simulink model "Tx_Rx"  (R2020a)
settings: Solver=VariableStepAuto  StartTime=0.0  StopTime=640e-9  RelTol=1e-3
libraries: msbUtilities x102, simulink_extras x15, dspswit3 x4, dspsigops x2
(part 3 of 3)

== matlab function Tx_Rx/BER_calculator/PI&PS/Phase Interpolator/MATLAB Function ==
  data: LSB_4bit input; c0_0 output; clk_s1 input; clk_s3 input; c0_1 output; c1_0 output; c1_1 output; c2_0 output; c2_1 output; c3_0 output; c3_1 output; c4_0 output; c4_1 output; c5_0 output; c5_1 output; c6_0 output; c6_1 output; c7_0 output; c7_1 output; c8_0 output; c8_1 output; c9_0 output; c9_1 output; c10_0 output; c10_1 output; c11_0 output; c11_1 output; c12_0 output; c12_1 output; c13_0 output; c13_1 output; c14_0 output; c14_1 output; c15_0 output; c15_1 output
function [c0_0,c0_1,c1_0,c1_1,c2_0,c2_1,c3_0,c3_1,c4_0,c4_1,c5_0,c5_1,c6_0,c6_1,c7_0,c7_1,c8_0,c8_1,c9_0,c9_1,c10_0,c10_1,c11_0,c11_1,c12_0,c12_1,c13_0,c13_1,c14_0,c14_1,c15_0,c15_1] = phase_interpolator(LSB_4bit,clk_s1,clk_s3)
    switch LSB_4bit
        case 0
            c0_0 = clk_s1;
            c0_1 = clk_s3;
            c1_0 = 0;
            c1_1 = 0;
            c2_0 = 0;
            c2_1 = 0;
            c3_0 = 0;
            c3_1 = 0;
            c4_0 = 0;
            c4_1 = 0;
            c5_0 = 0;
            c5_1 = 0;
            c6_0 = 0;
            c6_1 = 0;
            c7_0 = 0;
            c7_1 = 0;
            c8_0 = 0;
            c8_1 = 0;
            c9_0 = 0;
            c9_1 = 0;
            c10_0 = 0;
            c10_1 = 0;
            c11_0 = 0;
            c11_1 = 0;
            c12_0 = 0;
            c12_1 = 0;
            c13_0 = 0;
            c13_1 = 0;
            c14_0 = 0;
            c14_1 = 0;
            c15_0 = 0;
            c15_1 = 0;
        case 1
            c0_0 = 0;
            c0_1 = 0;
            c1_0 = clk_s1;
            c1_1 = clk_s3;
            c2_0 = 0;
            c2_1 = 0;
            c3_0 = 0;
            c3_1 = 0;
            c4_0 = 0;
            c4_1 = 0;
            c5_0 = 0;
            c5_1 = 0;
            c6_0 = 0;
            c6_1 = 0;
            c7_0 = 0;
            c7_1 = 0;
            c8_0 = 0;
            c8_1 = 0;
            c9_0 = 0;
            c9_1 = 0;
            c10_0 = 0;
            c10_1 = 0;
            c11_0 = 0;
            c11_1 = 0;
            c12_0 = 0;
            c12_1 = 0;
            c13_0 = 0;
            c13_1 = 0;
            c14_0 = 0;
            c14_1 = 0;
            c15_0 = 0;
            c15_1 = 0;
        case 10
            c0_0 = 0;
            c0_1 = 0;
            c1_0 = 0;
            c1_1 = 0;
            c2_0 = clk_s1;
            c2_1 = clk_s3;
            c3_0 = 0;
            c3_1 = 0;
            c4_0 = 0;
            c4_1 = 0;
            c5_0 = 0;
            c5_1 = 0;
            c6_0 = 0;
            c6_1 = 0;
            c7_0 = 0;
            c7_1 = 0;
            c8_0 = 0;
            c8_1 = 0;
            c9_0 = 0;
            c9_1 = 0;
            c10_0 = 0;
            c10_1 = 0;
            c11_0 = 0;
            c11_1 = 0;
            c12_0 = 0;
            c12_1 = 0;
            c13_0 = 0;
            c13_1 = 0;
            c14_0 = 0;
            c14_1 = 0;
            c15_0 = 0;
            c15_1 = 0;
        case 11
            c0_0 = 0;
            c0_1 = 0;
            c1_0 = 0;
            c1_1 = 0;
            c2_0 = 0;
            c2_1 = 0;
            c3_0 = clk_s1;
            c3_1 = clk_s3;
            c4_0 = 0;
            c4_1 = 0;
            c5_0 = 0;
            c5_1 = 0;
            c6_0 = 0;
            c6_1 = 0;
            c7_0 = 0;
            c7_1 = 0;
            c8_0 = 0;
            c8_1 = 0;
            c9_0 = 0;
            c9_1 = 0;
            c10_0 = 0;
            c10_1 = 0;
            c11_0 = 0;
            c11_1 = 0;
            c12_0 = 0;
            c12_1 = 0;
            c13_0 = 0;
            c13_1 = 0;
            c14_0 = 0;
            c14_1 = 0;
            c15_0 = 0;
            c15_1 = 0;
        case 100
            c0_0 = 0;
            c0_1 = 0;
            c1_0 = 0;
            c1_1 = 0;
            c2_0 = 0;
            c2_1 = 0;
            c3_0 = 0;
            c3_1 = 0;
            c4_0 = clk_s1;
            c4_1 = clk_s3;
            c5_0 = 0;
            c5_1 = 0;
            c6_0 = 0;
            c6_1 = 0;
            c7_0 = 0;
            c7_1 = 0;
            c8_0 = 0;
            c8_1 = 0;
            c9_0 = 0;
            c9_1 = 0;
            c10_0 = 0;
            c10_1 = 0;
            c11_0 = 0;
            c11_1 = 0;
            c12_0 = 0;
            c12_1 = 0;
            c13_0 = 0;
            c13_1 = 0;
            c14_0 = 0;
            c14_1 = 0;
            c15_0 = 0;
            c15_1 = 0;
        case 101
            c0_0 = 0;
            c0_1 = 0;
            c1_0 = 0;
            c1_1 = 0;
            c2_0 = 0;
            c2_1 = 0;
            c3_0 = 0;
            c3_1 = 0;
            c4_0 = 0;
            c4_1 = 0;
            c5_0 = clk_s1;
            c5_1 = clk_s3;
            c6_0 = 0;
            c6_1 = 0;
            c7_0 = 0;
            c7_1 = 0;
            c8_0 = 0;
            c8_1 = 0;
            c9_0 = 0;
            c9_1 = 0;
            c10_0 = 0;
            c10_1 = 0;
            c11_0 = 0;
            c11_1 = 0;
            c12_0 = 0;
            c12_1 = 0;
            c13_0 = 0;
            c13_1 = 0;
            c14_0 = 0;
            c14_1 = 0;
            c15_0 = 0;
            c15_1 = 0;
        case 110
            c0_0 = 0;
            c0_1 = 0;
            c1_0 = 0;
            c1_1 = 0;
            c2_0 = 0;
            c2_1 = 0;
            c3_0 = 0;
            c3_1 = 0;
            c4_0 = 0;
            c4_1 = 0;
            c5_0 = 0;
            c5_1 = 0;
            c6_0 = clk_s1;
            c6_1 = clk_s3;
            c7_0 = 0;
            c7_1 = 0;
            c8_0 = 0;
            c8_1 = 0;
            c9_0 = 0;
            c9_1 = 0;
            c10_0 = 0;
            c10_1 = 0;
            c11_0 = 0;
            c11_1 = 0;
            c12_0 = 0;
            c12_1 = 0;
            c13_0 = 0;
            c13_1 = 0;
            c14_0 = 0;
            c14_1 = 0;
            c15_0 = 0;
            c15_1 = 0;
        case 111
            c0_0 = 0;
            c0_1 = 0;
            c1_0 = 0;
            c1_1 = 0;
            c2_0 = 0;
            c2_1 = 0;
            c3_0 = 0;
            c3_1 = 0;
            c4_0 = 0;
            c4_1 = 0;
            c5_0 = 0;
            c5_1 = 0;
            c6_0 = 0;
            c6_1 = 0;
            c7_0 = clk_s1;
            c7_1 = clk_s3;
            c8_0 = 0;
            c8_1 = 0;
            c9_0 = 0;
            c9_1 = 0;
            c10_0 = 0;
            c10_1 = 0;
            c11_0 = 0;
            c11_1 = 0;
            c12_0 = 0;
            c12_1 = 0;
            c13_0 = 0;
            c13_1 = 0;
            c14_0 = 0;
            c14_1 = 0;
            c15_0 = 0;
            c15_1 = 0;
        case 1000
            c0_0 = 0;
            c0_1 = 0;
            c1_0 = 0;
            c1_1 = 0;
            c2_0 = 0;
            c2_1 = 0;
            c3_0 = 0;
            c3_1 = 0;
            c4_0 = 0;
            c4_1 = 0;
            c5_0 = 0;
            c5_1 = 0;
            c6_0 = 0;
            c6_1 = 0;
            c7_0 = 0;
            c7_1 = 0;
            c8_0 = clk_s1;
            c8_1 = clk_s3;
            c9_0 = 0;
            c9_1 = 0;
            c10_0 = 0;
            c10_1 = 0;
            c11_0 = 0;
            c11_1 = 0;
            c12_0 = 0;
            c12_1 = 0;
            c13_0 = 0;
            c13_1 = 0;
            c14_0 = 0;
            c14_1 = 0;
            c15_0 = 0;
            c15_1 = 0;
        case 1001
            c0_0 = 0;
            c0_1 = 0;
            c1_0 = 0;
            c1_1 = 0;
            c2_0 = 0;
            c2_1 = 0;
            c3_0 = 0;
            c3_1 = 0;
            c4_0 = 0;
            c4_1 = 0;
            c5_0 = 0;
            c5_1 = 0;
            c6_0 = 0;
            c6_1 = 0;
            c7_0 = 0;
            c7_1 = 0;
            c8_0 = 0;
            c8_1 = 0;
            c9_0 = clk_s1;
            c9_1 = clk_s3;
            c10_0 = 0;
            c10_1 = 0;
            c11_0 = 0;
            c11_1 = 0;
            c12_0 = 0;
            c12_1 = 0;
            c13_0 = 0;
            c13_1 = 0;
            c14_0 = 0;
            c14_1 = 0;
            c15_0 = 0;
            c15_1 = 0;
        case 1010
            c0_0 = 0;
            c0_1 = 0;
            c1_0 = 0;
            c1_1 = 0;
            c2_0 = 0;
            c2_1 = 0;
            c3_0 = 0;
            c3_1 = 0;
            c4_0 = 0;
            c4_1 = 0;
            c5_0 = 0;
            c5_1 = 0;
            c6_0 = 0;
            c6_1 = 0;
            c7_0 = 0;
            c7_1 = 0;
            c8_0 = 0;
            c8_1 = 0;
            c9_0 = 0;
            c9_1 = 0;
            c10_0 = clk_s1;
            c10_1 = clk_s3;
            c11_0 = 0;
            c11_1 = 0;
            c12_0 = 0;
            c12_1 = 0;
            c13_0 = 0;
            c13_1 = 0;
            c14_0 = 0;
            c14_1 = 0;
            c15_0 = 0;
            c15_1 = 0;   
        case 1011
            c0_0 = 0;
            c0_1 = 0;
            c1_0 = 0;
            c1_1 = 0;
            c2_0 = 0;
            c2_1 = 0;
            c3_0 = 0;
            c3_1 = 0;
            c4_0 = 0;
            c4_1 = 0;
            c5_0 = 0;
            c5_1 = 0;
            c6_0 = 0;
            c6_1 = 0;
            c7_0 = 0;
            c7_1 = 0;
            c8_0 = 0;
            c8_1 = 0;
            c9_0 = 0;
            c9_1 = 0;
            c10_0 = 0;
            c10_1 = 0;
            c11_0 = clk_s1;
            c11_1 = clk_s3;
            c12_0 = 0;
            c12_1 = 0;
            c13_0 = 0;
            c13_1 = 0;
            c14_0 = 0;
            c14_1 = 0;
            c15_0 = 0;
            c15_1 = 0;
        case 1100
            c0_0 = 0;
            c0_1 = 0;
            c1_0 = 0;
            c1_1 = 0;
            c2_0 = 0;
            c2_1 = 0;
            c3_0 = 0;
            c3_1 = 0;
            c4_0 = 0;
            c4_1 = 0;
            c5_0 = 0;
            c5_1 = 0;
            c6_0 = 0;
            c6_1 = 0;
            c7_0 = 0;
            c7_1 = 0;
            c8_0 = 0;
            c8_1 = 0;
            c9_0 = 0;
            c9_1 = 0;
            c10_0 = 0;
            c10_1 = 0;
            c11_0 = 0;
            c11_1 = 0;
            c12_0 = clk_s1;
            c12_1 = clk_s3;
            c13_0 = 0;
            c13_1 = 0;
            c14_0 = 0;
            c14_1 = 0;
            c15_0 = 0;
            c15_1 = 0;
        case 1101
            c0_0 = 0;
            c0_1 = 0;
            c1_0 = 0;
            c1_1 = 0;
            c2_0 = 0;
            c2_1 = 0;
            c3_0 = 0;
            c3_1 = 0;
            c4_0 = 0;
            c4_1 = 0;
            c5_0 = 0;
            c5_1 = 0;
            c6_0 = 0;
            c6_1 = 0;
            c7_0 = 0;
            c7_1 = 0;
            c8_0 = 0;
            c8_1 = 0;
            c9_0 = 0;
            c9_1 = 0;
            c10_0 = 0;
            c10_1 = 0;
            c11_0 = 0;
            c11_1 = 0;
            c12_0 = 0;
            c12_1 = 0;
            c13_0 = clk_s1;
            c13_1 = clk_s3;
            c14_0 = 0;
            c14_1 = 0;
            c15_0 = 0;
            c15_1 = 0;
        case 1110
            c0_0 = 0;
            c0_1 = 0;
            c1_0 = 0;
            c1_1 = 0;
            c2_0 = 0;
            c2_1 = 0;
            c3_0 = 0;
            c3_1 = 0;
            c4_0 = 0;
            c4_1 = 0;
            c5_0 = 0;
            c5_1 = 0;
            c6_0 = 0;
            c6_1 = 0;
            c7_0 = 0;
            c7_1 = 0;
            c8_0 = 0;
            c8_1 = 0;
            c9_0 = 0;
            c9_1 = 0;
            c10_0 = 0;
            c10_1 = 0;
            c11_0 = 0;
            c11_1 = 0;
            c12_0 = 0;
            c12_1 = 0;
            c13_0 = 0;
            c13_1 = 0;
            c14_0 = clk_s1;
            c14_1 = clk_s3;
            c15_0 = 0;
            c15_1 = 0;
        otherwise
            c0_0 = 0;
            c0_1 = 0;
            c1_0 = 0;
            c1_1 = 0;
            c2_0 = 0;
            c2_1 = 0;
            c3_0 = 0;
            c3_1 = 0;
            c4_0 = 0;
            c4_1 = 0;
            c5_0 = 0;
            c5_1 = 0;
            c6_0 = 0;
            c6_1 = 0;
            c7_0 = 0;
            c7_1 = 0;
            c8_0 = 0;
            c8_1 = 0;
            c9_0 = 0;
            c9_1 = 0;
            c10_0 = 0;
            c10_1 = 0;
            c11_0 = 0;
            c11_1 = 0;
            c12_0 = 0;
            c12_1 = 0;
            c13_0 = 0;
            c13_1 = 0;
            c14_0 = 0;
            c14_1 = 0;
            c15_0 = clk_s1;
            c15_1 = clk_s3;
    end
